simulink model "MotorDriveUnit_harness_model"  (R2022a)
settings: Solver=daessc  StartTime=0.0  StopTime=10.0  RelTol=1e-3
PreLoadFcn:
  | BEV_params
libraries: fl_lib x12, nesl_utility x5, sdl_lib x1
settings Model: Creator=isaacito  LastModifiedBy=isaacito
settings DataIOCC: DSMLogging=off
settings SimscapeCC: SimscapeLogType=all  SimscapeLogSimulationStatistics=on  SimscapeLogLimitData=off

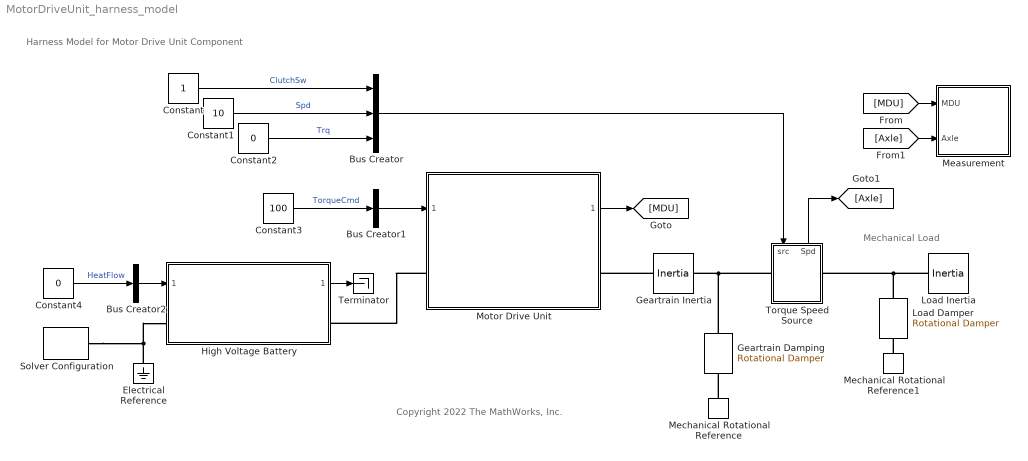
== system MotorDriveUnit_harness_model ==
  note: Mechanical Load
  note: Harness Model for Motor Drive Unit Component
  note: Copyright 2022 The MathWorks, Inc.
  Bus Creator : BusCreator  Inputs=3
  Bus Creator1 : BusCreator  Inputs=1
  Bus Creator2 : BusCreator  Inputs=1
  Constant : Constant
  Constant1 : Constant  Value=10
  Constant2 : Constant  Value=0
  Constant3 : Constant  Value=100
  Constant4 : Constant  Value=0
  Electrical Reference : fl_lib/Electrical/Electrical Elements/Electrical Reference
      settings: SourceProductBaseCode=PW,SS,VE
  Geartrain Damping : fl_lib/Mechanical/Rotational Elements/Rotational Damper  D=0.001 m*N/rpm  w_specify=off  w_priority=None  w=0 rad/s  w_nominal_specify=off  w_nominal_unit=rad/s  w_nominal_value=1  t_specify=off  t_priority=None  t=0 N*m  t_nominal_specify=off  t_nominal_unit=N*m  t_nominal_value=1
      settings: SourceProductBaseCode=PW,SS,VE
      settings: AttributesFormatString=|
      | %<D>
      | %<D_unit>
  Geartrain Inertia : fl_lib/Mechanical/Rotational Elements/Inertia  inertia=15*0.3^2 kg*m^2  num_ports=foundation.enum.numPorts2.two  w_specify=on  w_priority=None  w=0 rpm  w_nominal_specify=off  w_nominal_unit=rad/s  w_nominal_value=1  t_specify=off  t_priority=None  t=0 N*m  t_nominal_specify=off  t_nominal_unit=N*m  t_nominal_value=1
      settings: SourceProductBaseCode=PW,SS,VE  InternalSimscapePortConfiguration="{\"Bottom\":[],\"Left\":[{\"id\":\"I\",\"label\":\"\",\"type\":\"foundation.mechanical.rotational.rotational\"}],\"Right\":[{\"id\":\"J\",\"label\":\"\",\"type\":\"foundation.mechanical.rotational.rotational\"}],\"Top\":[]}"
      settings: AttributesFormatString=|
      | %<inertia>
      | %<inertia_unit>
  High Voltage Battery : Subsystem  ReferencedSubsystem=BatteryHV_refsub_Basic
  Load Damper : fl_lib/Mechanical/Rotational Elements/Rotational Damper  D=0.1 N*m/rpm  w_specify=off  w_priority=None  w=0 rad/s  w_nominal_specify=off  w_nominal_unit=rad/s  w_nominal_value=1  t_specify=off  t_priority=None  t=0 N*m  t_nominal_specify=off  t_nominal_unit=N*m  t_nominal_value=1
      settings: SourceProductBaseCode=PW,SS,VE
  Load Inertia : fl_lib/Mechanical/Rotational Elements/Inertia  inertia=2000*0.3^3 kg*m^2  num_ports=foundation.enum.numPorts2.one  w_specify=off  w_priority=High  w=0 rad/s  w_nominal_specify=off  w_nominal_unit=rad/s  w_nominal_value=1  t_specify=off  t_priority=None  t=0 N*m  t_nominal_specify=off  t_nominal_unit=N*m  t_nominal_value=1
      settings: SourceProductBaseCode=PW,SS,VE
  Measurement : Subsystem
  Mechanical Rotational Reference : fl_lib/Mechanical/Rotational Elements/Mechanical Rotational Reference
      settings: SourceProductBaseCode=PW,SS,VE
  Mechanical Rotational Reference1 : fl_lib/Mechanical/Rotational Elements/Mechanical Rotational Reference
      settings: SourceProductBaseCode=PW,SS,VE
  Motor Drive Unit : Subsystem  ReferencedSubsystem=MotorDriveUnit_refsub_Basic
  Solver Configuration : nesl_utility/Solver Configuration  PhysicalDomain=network_engine_domain  SubClassName=solver  LeftPortType=input  RightPortType=generic  Tones=[]  Harmonics=[]  SimulateNoise=off  Profile=off  UseLocalSampling=off  EnableSwitchedLinearOptims=on  FrequencyDomain=off  UseCCode=off  RelTol=0.001  AbsTol=1e-06  MinStep=1e-09  ToWorkspace=off  RevertToSquareIcSolve=off  NumHomotopyIterations=100  PhasorMode=off  PhasorModeNumHarmonics=1  IndexReductionMethod=DerivativeReplacement  DoDC=off  ResidualTolerance=1e-09  UseLocalSolver=off  LocalSolverChoice=NE_BACKWARD_EULER_ADVANCER  LocalSolverSampleTime=0.001  DoFixedCost=off  MaxNonlinIter=3  MaxModeIter=2  ComputeImpulses=off  ImpulseIterations=2  LinearAlgebra=auto  LinearAlgebraNumThread=0  EquationFormulation=NE_TIME_EF  DelaysMemoryBudget=1024  AutomaticFiltering=on  FilteringTimeConstant=0.001  PartitionStorageMethod=AS_NEEDED  PartitionMemoryBudget=1024  PartitionMethod=ROBUST
      settings: AttributesFormatString=Local solver %<UseLocalSolver>  SourceProductBaseCode=SS,PW,VE
  Terminator : Terminator
  Torque Speed Source : Subsystem
      settings: PortSchema="{\"entries\":[{\"content\":{\"sides\":[{\"content\":{\"connectorIds\":[\"LConn1\"]},\"type\":\"ConnectorPlacement.EquallySpacedRectSide\",\"uuid\":\"92a06674-aaa2-495f-b380-fd1e5a218eb3\"},{\"content\":{\"connectorIds\":[\"RConn1\"],\"side\":\"RIGHT\"},\"type\":\"ConnectorPlacement.EquallySpacedRectSide\",\"uuid\":\"3e9807eb-b215-4ab1-ac02-6574a58f93c0\"},{\"content\":{\"connectorIds\":[\"In1\",\"Out1\"],\"side\":\"TOP\"},\"type\":\"ConnectorPlacement.EquallySpacedRectSide\",\"uuid\":\"937668c8-63b6-43a7-85c7-81bf7d359316\"}]},\"type\":\"ConnectorPlacement.EquallySpacedConnector\",\"uuid\":\"ba9b6e46-9639-4838-8d50-8636a64d3a24\"}],\"packageUris\":[\"http://schema.mathworks.com/mf0/Connector/R2020b\"],\"version\":\"1.0\"}"
  wires:
  Constant/1 -> Bus Creator/1  "ClutchSw"
  Constant1/1 -> Bus Creator/2  "Spd"
  Constant2/1 -> Bus Creator/3  "Trq"
  Bus Creator/1 -> Torque Speed Source/1(src)
  Motor Drive Unit/1 -> [MDU]
  [MDU] -> Measurement/1(MDU)
  Constant3/1 -> Bus Creator1/1  "TorqueCmd"
  Bus Creator1/1 -> Motor Drive Unit/1
  Torque Speed Source/1(Spd) -> [Axle]
  [Axle] -> Measurement/2(Axle)
  Constant4/1 -> Bus Creator2/1  "HeatFlow"
  Bus Creator2/1 -> High Voltage Battery/1
  High Voltage Battery/1 -> Terminator/1
  connections:
  Geartrain Inertia/RConn1 -- Motor Drive Unit/RConn1
  Mechanical Rotational Reference/LConn1 -- Geartrain Damping/RConn1
  Torque Speed Source/LConn1 -- Geartrain Damping/LConn1 -- Geartrain Inertia/LConn1
  Load Inertia/LConn1 -- Torque Speed Source/RConn1 -- Load Damper/LConn1
  Mechanical Rotational Reference1/LConn1 -- Load Damper/RConn1
  Motor Drive Unit/LConn1 -- High Voltage Battery/RConn1
  Electrical Reference/LConn1 -- Solver Configuration/RConn1 -- High Voltage Battery/LConn1

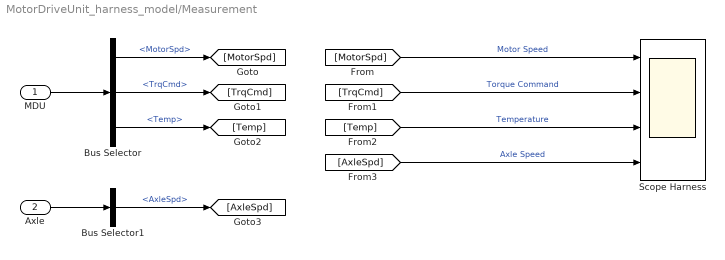
== system MotorDriveUnit_harness_model/Measurement ==
  MDU : Inport
  Axle : Inport  Port=2
  Bus Selector : BusSelector  OutputSignals=MotorSpd,TrqCmd,Temp
  Bus Selector1 : BusSelector  OutputSignals=AxleSpd
  Scope Harness : Scope  NumInputPorts=4
  wires:
  MDU/1 -> Bus Selector/1
  Bus Selector/1 -> [MotorSpd]  "<MotorSpd>"
  Bus Selector/2 -> [TrqCmd]  "<TrqCmd>"
  Bus Selector/3 -> [Temp]  "<Temp>"
  [MotorSpd] -> Scope Harness/1  "Motor Speed"
  [TrqCmd] -> Scope Harness/2  "Torque Command"
  [Temp] -> Scope Harness/3  "Temperature"
  Axle/1 -> Bus Selector1/1
  Bus Selector1/1 -> [AxleSpd]  "<AxleSpd>"
  [AxleSpd] -> Scope Harness/4  "Axle Speed"

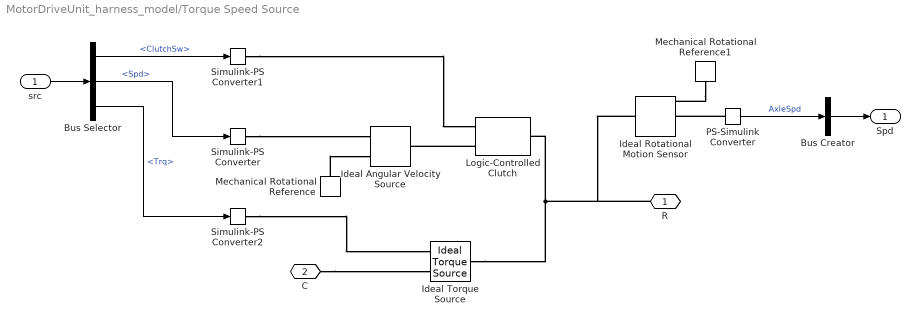
== system MotorDriveUnit_harness_model/Torque Speed Source ==
  src : Inport
  Bus Creator : BusCreator  Inputs=1
  Bus Selector : BusSelector  OutputSignals=ClutchSw,Spd,Trq
  Ideal Angular Velocity Source : fl_lib/Mechanical/Mechanical Sources/Ideal Angular Velocity Source
      settings: SourceProductBaseCode=PW,SS,VE
  Ideal Rotational Motion Sensor : fl_lib/Mechanical/Mechanical Sensors/Ideal Rotational Motion Sensor  wrap_angle=simscape.enum.onoff.off  offset=0 rad
      settings: SourceProductBaseCode=PW,SS,VE
  Ideal Torque Source : fl_lib/Mechanical/Mechanical Sources/Ideal Torque Source
      settings: SourceProductBaseCode=PW,SS,VE
  Logic-Controlled Clutch : sdl_lib/Clutches/Logic-Controlled Clutch  transition_model=sdl.enum.transitionModel.instant  transition_time_constant=0.1 s  t_friction=5000 N*m  t_locked=5000 N*m  w_tol=0.1 rpm  initial_state_locked=sdl.enum.initial_lock.unlocked
      settings: SourceProductBaseCode=LD  InternalSimscapePortConfiguration="{\"Bottom\":[],\"Left\":[{\"id\":\"E\",\"label\":\"E\",\"type\":\"input\"},{\"id\":\"B\",\"label\":\"B\",\"type\":\"foundation.mechanical.rotational.rotational\"}],\"Right\":[{\"id\":\"F\",\"label\":\"F\",\"type\":\"foundation.mechanical.rotational.rotational\"}],\"Top\":[]}"
  Mechanical Rotational Reference : fl_lib/Mechanical/Rotational Elements/Mechanical Rotational Reference
      settings: SourceProductBaseCode=PW,SS,VE
  Mechanical Rotational Reference1 : fl_lib/Mechanical/Rotational Elements/Mechanical Rotational Reference
      settings: SourceProductBaseCode=PW,SS,VE
  PS-Simulink Converter : nesl_utility/PS-Simulink Converter  PhysicalDomain=network_engine_domain  SubClassName=ps_output  LeftPortType=input  RightPortType=output  PseudoPeriodic=off  Frequencies=[]  VectorFormat=inherit  Unit=rpm  AffineConversion=off
      settings: SourceProductBaseCode=SS,PW,VE
  Simulink-PS Converter : nesl_utility/Simulink-PS Converter  PhysicalDomain=network_engine_domain  SubClassName=ps_input  LeftPortType=input  RightPortType=output  PseudoPeriodic=off  Frequencies=[]  NoiseDistribution=none  NoiseParameters=[]  Unit=rpm  AffineConversion=off  FilteringAndDerivatives=provide  SimscapeFilterOrder=1  InputFilterTimeConstant=0.001  UdotUserProvided=0
      settings: SourceProductBaseCode=SS,PW,VE
  Simulink-PS Converter1 : nesl_utility/Simulink-PS Converter  PhysicalDomain=network_engine_domain  SubClassName=ps_input  LeftPortType=input  RightPortType=output  PseudoPeriodic=off  Frequencies=[]  NoiseDistribution=none  NoiseParameters=[]  Unit=1  AffineConversion=off  FilteringAndDerivatives=zero  SimscapeFilterOrder=1  InputFilterTimeConstant=0.001  UdotUserProvided=0
      settings: SourceProductBaseCode=SS,PW,VE
      settings: AttributesFormatString=|
      | %<Unit>
      | Derivative: %<FilteringAndDerivatives>
  Simulink-PS Converter2 : nesl_utility/Simulink-PS Converter  PhysicalDomain=network_engine_domain  SubClassName=ps_input  LeftPortType=input  RightPortType=output  PseudoPeriodic=off  Frequencies=[]  NoiseDistribution=none  NoiseParameters=[]  Unit=N*m  AffineConversion=off  FilteringAndDerivatives=provide  SimscapeFilterOrder=1  InputFilterTimeConstant=0.001  UdotUserProvided=0
      settings: SourceProductBaseCode=SS,PW,VE
  R : PMIOPort  Side=Left
  C : PMIOPort  Port=2  Side=Right
  Spd : Outport
  wires:
  src/1 -> Bus Selector/1
  Bus Selector/1 -> Simulink-PS Converter1/1  "<ClutchSw>"
  Bus Selector/2 -> Simulink-PS Converter/1  "<Spd>"
  Bus Selector/3 -> Simulink-PS Converter2/1  "<Trq>"
  PS-Simulink Converter/1 -> Bus Creator/1  "AxleSpd"
  Bus Creator/1 -> Spd/1
  connections:
  Simulink-PS Converter/RConn1 -- Ideal Angular Velocity Source/RConn1
  Mechanical Rotational Reference/LConn1 -- Ideal Angular Velocity Source/RConn2
  Logic-Controlled Clutch/LConn2 -- Ideal Angular Velocity Source/LConn1
  Simulink-PS Converter1/RConn1 -- Logic-Controlled Clutch/LConn1
  Simulink-PS Converter2/RConn1 -- Ideal Torque Source/RConn1
  Ideal Torque Source/LConn1 -- Ideal Rotational Motion Sensor/LConn1 -- R/RConn1 -- Logic-Controlled Clutch/RConn1
  C/RConn1 -- Ideal Torque Source/RConn2
  Mechanical Rotational Reference1/LConn1 -- Ideal Rotational Motion Sensor/RConn1
  PS-Simulink Converter/LConn1 -- Ideal Rotational Motion Sensor/RConn2
